simulink library "motor_feedback"  (R2018a)
settings: Solver=VariableStepAuto  StartTime=0.0  StopTime=10.0  RelTol=1e-3
values from neighbouring files (symbols this model uses):
  motorFeedback = Feedback.MotorFeedback(stanceLeft,stanceRight,swingLeft,swingRight)    [soccer_strategy_setup.m]
undefined symbols (not defined in the file or in its folder): DiscIntNeverNeededParam
libraries: simulink x1
settings Model: Creator=daniel  LastModifiedBy=vuwij

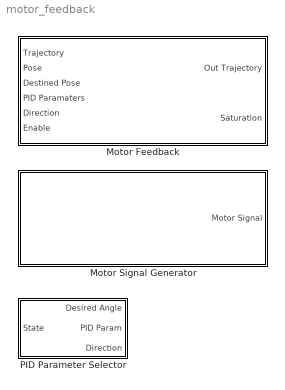
== system motor_feedback ==
  Motor Feedback : Subsystem  mask{motorNumber=1, upperLimit=0.1, lowerLimit=-0.1, reverseDirection=on}
      mask prompts: motorNumber "Motor Number:"; upperLimit "Upper Limit:"; lowerLimit "Lower Limit:"; reverseDirection "Reverse Direction"
  Motor Signal Generator : Subsystem
  PID Parameter Selector : Subsystem  mask{pidParamSet=motorFeedback.rightHipSideFront.pitch, angleParamSet=motorFeedback.desiredAngle.pitch}
      mask prompts: pidParamSet "PID Parameter Set:"; angleParamSet "Angle Parameter Set:"

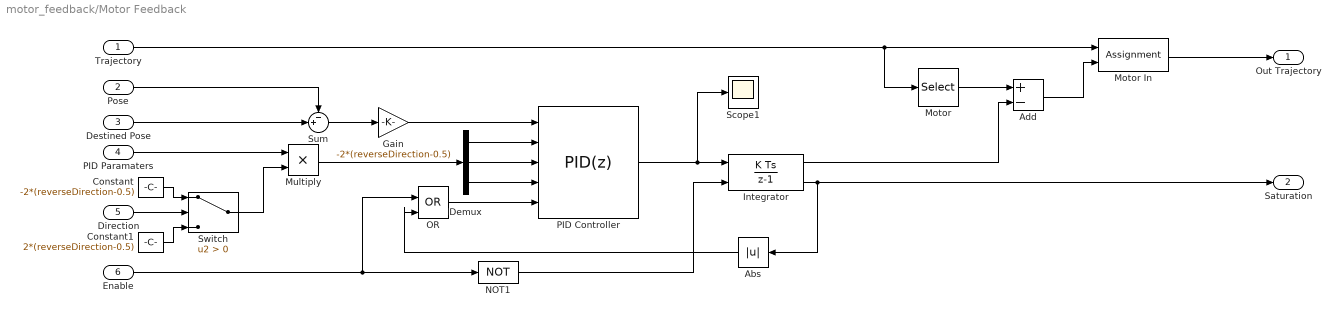
== system motor_feedback/Motor Feedback ==
  Trajectory : Inport
  Pose : Inport  Port=2
  Destined Pose : Inport  Port=3
  PID Paramaters : Inport  Port=4
  Direction : Inport  Port=5
  Enable : Inport  Port=6
  Abs : Abs
  Add : Sum  Inputs=+-
  Constant : Constant  Value=-2*(reverseDirection-0.5)
  Constant1 : Constant  Value=2*(reverseDirection-0.5)
  Demux : Demux  Outputs=3
  Gain : Gain  Gain=-2*(reverseDirection-0.5)
  Integrator : DiscreteIntegrator  gainval=1  ExternalReset=level  SampleTime=-1  LimitOutput=on  UpperSaturationLimit=upperLimit  LowerSaturationLimit=lowerLimit  ShowSaturationPort=on  ICPrevOutput=DiscIntNeverNeededParam  ICPrevScaledInput=DiscIntNeverNeededParam
  Motor : Selector  InputPortWidth=20  IndexOptions=Index vector (dialog)  Indices=motorNumber  OutputSizes=1
  Motor In : Assignment  DiagnosticForDimensions=Warning  IndexOptions=Index vector (dialog)  Indices=motorNumber  OutputSizes=1
  Multiply : Product
  NOT1 : Logic  Operator=NOT  IconShape=distinctive  AllPortsSameDT=off  OutDataTypeStr=boolean
  OR : Logic  Operator=OR  IconShape=distinctive  AllPortsSameDT=off  OutDataTypeStr=boolean
  PID Controller : simulink/Continuous/PID Controller  Controller=PID  TimeDomain=Discrete-time  SampleTime=-1  IntegratorMethod=Forward Euler  FilterMethod=Forward Euler  Form=Parallel  UseFilter=off  ControllerParametersSource=external  P=0.5  I=1  D=0.001  N=100  InitialConditionSource=internal  InitialConditionForIntegrator=0  InitialConditionForFilter=0  ExternalReset=level  LimitOutput=off  UpperSaturationLimit=inf  LowerSaturationLimit=-inf  LinearizeAsGain=on  AntiWindupMode=none  Kb=1  TrackingMode=off  Kt=1  PParamMin=[]  PParamMax=[]  IParamMin=[]  IParamMax=[]  DParamMin=[]  DParamMax=[]  NParamMin=[]  NParamMax=[]  KbParamMin=[]  KbParamMax=[]  KtParamMin=[]  KtParamMax=[]  POutMin=[]  POutMax=[]  IOutMin=[]  IOutMax=[]  DOutMin=[]  DOutMax=[]  NOutMin=[]  NOutMax=[]  KbOutMin=[]  KbOutMax=[]  KtOutMin=[]  KtOutMax=[]  IntegratorOutMin=[]  IntegratorOutMax=[]  FilterOutMin=[]  FilterOutMax=[]  SumOutMin=[]  SumOutMax=[]  SumI1OutMin=[]  SumI1OutMax=[]  SumI2OutMin=[]  SumI2OutMax=[]  SumI3OutMin=[]  SumI3OutMax=[]  SumDOutMin=[]  SumDOutMax=[]  SaturationOutMin=[]  SaturationOutMax=[]  IntegratorContinuousStateAttributes=''  IntegratorStateMustResolveToSignalObject=off  IntegratorRTWStateStorageClass=Auto  FilterContinuousStateAttributes=''  FilterStateMustResolveToSignalObject=off  FilterRTWStateStorageClass=Auto  DifferentiatorICPrevScaledInput=0  DifferentiatorOutMin=[]  DifferentiatorOutMax=[]  FilterDiffOutCoefMin=[]  FilterDiffOutCoefMax=[]  SumDenOutMin=[]  SumDenOutMax=[]  SumNumOutMin=[]  SumNumOutMax=[]  ReciprocalOutMin=[]  ReciprocalOutMax=[]  DivideOutMin=[]  DivideOutMax=[]  TunerSelectOption=Transfer Function Based (PID Tuner App)
  Scope1 : Scope
  Sum : Sum  Inputs=-+|
  Switch : Switch  Criteria=u2 > Threshold
  Out Trajectory : Outport
  Saturation : Outport  Port=2
  wires:
  Sum/1 -> Gain/1
  Trajectory/1 -> Motor/1, Motor In/1
  Destined Pose/1 -> Sum/2
  Motor In/1 -> Out Trajectory/1
  Motor/1 -> Add/1
  Pose/1 -> Sum/1
  Add/1 -> Motor In/2
  Integrator/1 -> Add/2
  Multiply/1 -> Demux/1
  Demux/1 -> PID Controller/2
  Demux/3 -> PID Controller/4
  Demux/2 -> PID Controller/3
  PID Controller/1 -> Scope1/1, Integrator/1
  Enable/1 -> OR/1, NOT1/1
  OR/1 -> PID Controller/5
  Integrator/2 -> Abs/1, Saturation/1
  Gain/1 -> PID Controller/1
  NOT1/1 -> Integrator/2
  Abs/1 -> OR/2
  Direction/1 -> Switch/2
  Constant/1 -> Switch/1
  Constant1/1 -> Switch/3
  PID Paramaters/1 -> Multiply/1
  Switch/1 -> Multiply/2

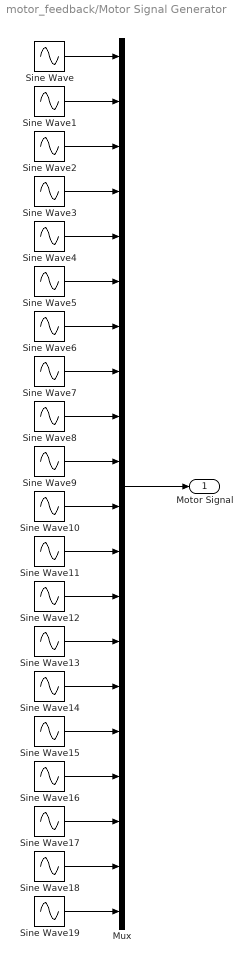
== system motor_feedback/Motor Signal Generator ==
  Mux : Mux  Inputs=20
  Sine Wave{,1..19} (20 alike) : Sin  SampleTime=0
  Motor Signal : Outport
  wires:
  Sine Wave2/1 -> Mux/3
  Sine Wave3/1 -> Mux/4
  Sine Wave10/1 -> Mux/11
  Mux/1 -> Motor Signal/1
  Sine Wave12/1 -> Mux/13
  Sine Wave7/1 -> Mux/8
  Sine Wave18/1 -> Mux/19
  Sine Wave19/1 -> Mux/20
  Sine Wave9/1 -> Mux/10
  Sine Wave4/1 -> Mux/5
  Sine Wave8/1 -> Mux/9
  Sine Wave13/1 -> Mux/14
  Sine Wave15/1 -> Mux/16
  Sine Wave17/1 -> Mux/18
  Sine Wave11/1 -> Mux/12
  Sine Wave14/1 -> Mux/15
  Sine Wave6/1 -> Mux/7
  Sine Wave16/1 -> Mux/17
  Sine Wave1/1 -> Mux/2
  Sine Wave/1 -> Mux/1
  Sine Wave5/1 -> Mux/6

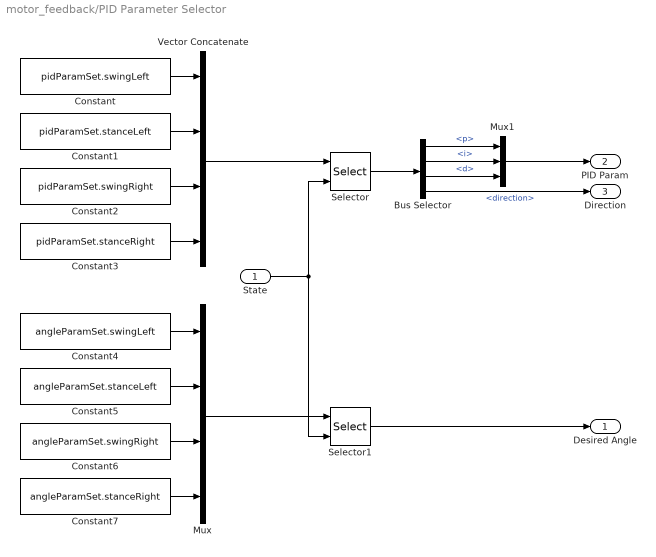
== system motor_feedback/PID Parameter Selector ==
  State : Inport  OutMin=1
  Bus Selector : BusSelector  OutputSignals=p,i,d,direction
  Constant : Constant  Value=pidParamSet.swingLeft  OutDataTypeStr=Bus: pid_values
  Constant1 : Constant  Value=pidParamSet.stanceLeft  OutDataTypeStr=Bus: pid_values
  Constant2 : Constant  Value=pidParamSet.swingRight  OutDataTypeStr=Bus: pid_values
  Constant3 : Constant  Value=pidParamSet.stanceRight  OutDataTypeStr=Bus: pid_values
  Constant4 : Constant  Value=angleParamSet.swingLeft  OutDataTypeStr=double
  Constant5 : Constant  Value=angleParamSet.stanceLeft  OutDataTypeStr=double
  Constant6 : Constant  Value=angleParamSet.swingRight  OutDataTypeStr=double
  Constant7 : Constant  Value=angleParamSet.stanceRight  OutDataTypeStr=double
  Mux : Mux
  Mux1 : Mux  Inputs=3
  Selector : Selector  InputPortWidth=4  IndexOptions=Index vector (port)  Indices=[1 3]  OutputSizes=1
  Selector1 : Selector  InputPortWidth=4  IndexOptions=Index vector (port)  Indices=[1 3]  OutputSizes=1
  Vector Concatenate : Concatenate  NumInputs=4
  Desired Angle : Outport
  PID Param : Outport  Port=2
  Direction : Outport  Port=3
  wires:
  Constant1/1 -> Vector Concatenate/2
  Mux1/1 -> PID Param/1
  Bus Selector/1 -> Mux1/1  "<p>"
  Bus Selector/2 -> Mux1/2  "<i>"
  Bus Selector/3 -> Mux1/3  "<d>"
  Constant/1 -> Vector Concatenate/1
  Bus Selector/4 -> Direction/1  "<direction>"
  Selector/1 -> Bus Selector/1
  Constant2/1 -> Vector Concatenate/3
  Constant3/1 -> Vector Concatenate/4
  Vector Concatenate/1 -> Selector/1
  Constant5/1 -> Mux/2
  Constant4/1 -> Mux/1
  State/1 -> Selector/2, Selector1/2
  Selector1/1 -> Desired Angle/1
  Mux/1 -> Selector1/1
  Constant7/1 -> Mux/4
  Constant6/1 -> Mux/3
